simulink model "double_luenberger"  (R2015a)
settings: Solver=ode45  StartTime=0.0  StopTime=3  RelTol=1e-3
PreLoadFcn:
  | double_pend_feedback
InitFcn:
  | double_pend_feedback
StartFcn:
  | double_pend_feedback
values from neighbouring files (symbols this model uses):
  A = [zeros(3,3) eye(3); -inv(D_)*G zeros(3,3)]    [double_pend_feedback.m]    (also in fuzzy_logic.m = [zeros(3,3) eye(3); inv(D_)*G zeros(3,3)]; single_pend.m = [0 1 0 0; (g*(M+m))/(l*M) 0 0 b/(l*M); 0 0 0 1; -m*g/M 0 0 -)
  a = 0.1    [double_pend_feedback.m]    (also in fuzzy_logic.m; single_pend.m)
  A_ = [0 1 0 0; -k/mass -damper/mass (sqrt(ep*2*a*k))/ep*a*mass 0; 0 0 0 1; 0 0 0 -R/L]    [double_pend_feedback.m]    (also in fuzzy_logic.m; single_pend.m)
  B = [zeros(3,1); inv(D_)*H]    [double_pend_feedback.m]    (also in fuzzy_logic.m; single_pend.m = [0;-1/(l*M); 0 ; 1/M])
  B_ = [0; 1/mass; 0;0]    [double_pend_feedback.m]    (also in fuzzy_logic.m; single_pend.m)
  damper = 200    [double_pend_feedback.m]    (also in fuzzy_logic.m; single_pend.m)
  ep = 1    [double_pend_feedback.m]    (also in fuzzy_logic.m; single_pend.m)
  k = 1    [double_pend_feedback.m]    (also in fuzzy_logic.m; single_pend.m)
  K_confirm = acker(A,B,p)    [double_pend_feedback.m]    (also in fuzzy_logic.m)
  Ke_confirm = acker(A',C',pe)    [double_pend_feedback.m]    (also in fuzzy_logic.m)
  L = 0.0001    [double_pend_feedback.m]    (also in fuzzy_logic.m; single_pend.m)
  mass = 0.5    [double_pend_feedback.m]    (also in fuzzy_logic.m; single_pend.m)
  R = 100    [double_pend_feedback.m]    (also in fuzzy_logic.m; single_pend.m)
libraries: simulink x1
settings Model: Creator=Nabeel  LastModifiedBy=Nabeel

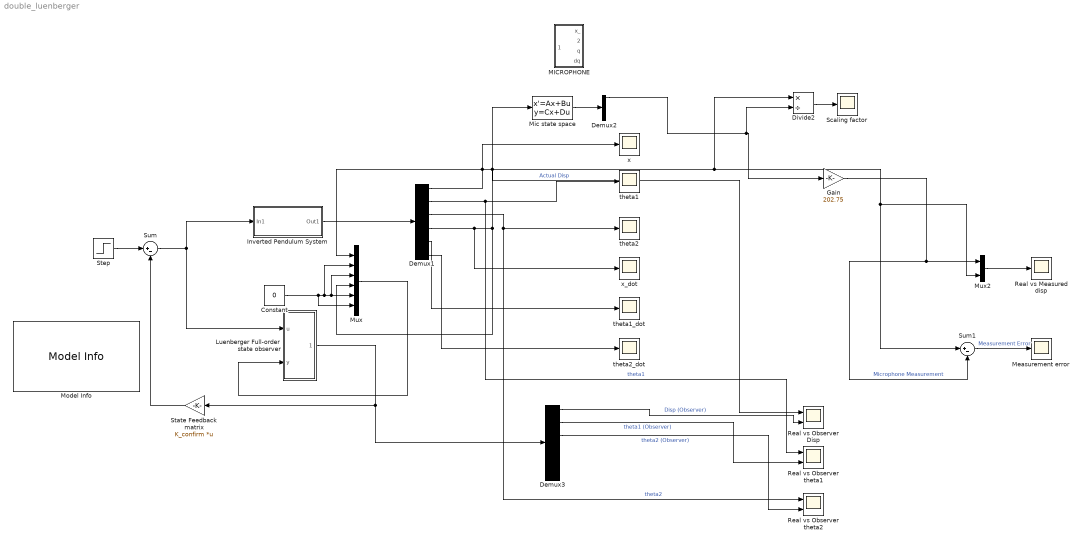
== system double_luenberger ==
  Constant : Constant  Value=0
  Demux1 : Demux  Outputs=6
  Demux2 : Demux
  Demux3 : Demux  Outputs=6
  Divide2 : Product  Inputs=*/
  Gain : Gain  Gain=202.75
  Inverted Pendulum System : Subsystem
  Luenberger Full-order state observer : Subsystem
  MICROPHONE : Subsystem
  Measurement error : Scope
      settings: ShowLegends=on  SaveName=error
  Mic state space : StateSpace  A=A_  B=B_  C=eye(4)  D=[0;0;0;0]  X0=0
  Model Info : simulink/Model-Wide Utilities/Model Info  Frame=on  DisplayStringWithTags=|  HorizontalTextAlignment=Center  LeftAlignmentValue=0.5  SourceBlockDiagram=double_luenberger  TagMaxNumber=20
      | State feedback matrix info:
      | Replace the feedback block
      |  to test other controllers
      | Gain block
      | K- pole placement (non-repeated)
      | lqr1 - LQR 1 as defined in report
      | lqr2- LQR 2 as defined in the report
  Mux : Mux  Inputs=6
  Mux2 : Mux  Inputs=2
  Real vs Measured disp : Scope
      settings: ShowLegends=on  SaveName=mic_v_real
  Real vs Observer Disp : Scope  NumInputPorts=2
      settings: ShowLegends=on  YMin=-425000~-5  YMax=75000~5  SaveName=results
  Real vs Observer theta1 : Scope  NumInputPorts=2
      settings: ShowLegends=on  YMin=-425000~-5  YMax=75000~5  SaveName=results1
  Real vs Observer theta2 : Scope  NumInputPorts=2
      settings: ShowLegends=on  YMin=-425000~-5  YMax=75000~5  SaveName=results2
  Scaling factor : Scope
      settings: ShowLegends=on  SaveName=scaling
  State Feedback matrix : Gain  Gain=K_confirm  Multiplication=Matrix(K*u)
  Step : Step  SampleTime=0
  Sum : Sum  Inputs=|+-
  Sum1 : Sum  Inputs=|+-
  theta1 : Scope
      settings: SaveName=theta1
  theta1_dot : Scope
      settings: SaveName=theta1_dot
  theta2 : Scope
      settings: SaveName=theta2
  theta2_dot : Scope
      settings: SaveName=theta2_dot
  x : Scope
      settings: SaveName=x
  x_dot : Scope
      settings: SaveName=x_dot
  wires:
  Inverted Pendulum System/1(Out1) -> Demux1/1
  Constant/1 -> Mux/6, Mux/2, Mux/3, Mux/5
  Mux/1 -> Luenberger Full-order state observer/2(y)
  Demux1/2 -> theta1/1, Real vs Observer theta1/1  "theta1"
  Demux1/1 -> x/1, Divide2/1, Sum1/1, Mux2/2, Real vs Observer Disp/1, Mux/1  "Actual Disp"
  Mic state space/1 -> Demux2/1
  Step/1 -> Sum/1
  State Feedback matrix/1 -> Sum/2
  Sum/1 -> Inverted Pendulum System/1(In1), Luenberger Full-order state observer/1(u)
  Luenberger Full-order state observer/1(x_estimate) -> Demux3/1, State Feedback matrix/1
  Demux3/1 -> Real vs Observer Disp/2  "Disp (Observer)"
  Demux3/2 -> Real vs Observer theta1/2  "theta1 (Observer)"
  Demux3/3 -> Real vs Observer theta2/2  "theta2 (Observer)"
  Demux1/3 -> theta2/1, Real vs Observer theta2/1  "theta2"
  Gain/1 -> Mux2/1, Sum1/2  "Microphone Measurement"
  Mux2/1 -> Real vs Measured disp/1
  Sum1/1 -> Measurement error/1  "Measurement Error"
  Demux2/1 -> Divide2/2, Gain/1
  Divide2/1 -> Scaling factor/1
  Demux1/5 -> theta1_dot/1
  Demux1/6 -> theta2_dot/1
  Demux1/4 -> x_dot/1, Mic state space/1, Mux/4

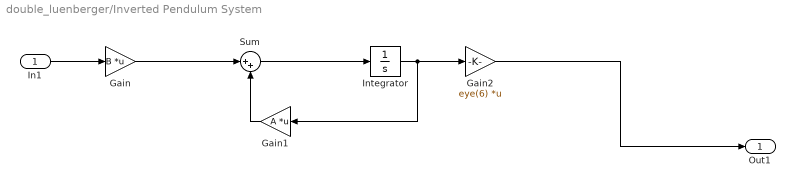
== system double_luenberger/Inverted Pendulum System ==
  In1 : Inport
  Gain : Gain  Gain=B  Multiplication=Matrix(K*u)
  Gain1 : Gain  Gain=A  Multiplication=Matrix(K*u)
  Gain2 : Gain  Gain=eye(6)  Multiplication=Matrix(K*u)
  Integrator : Integrator  InitialCondition=[0 0 0 0 0 0]
  Sum : Sum  Inputs=|++
  Out1 : Outport
  wires:
  In1/1 -> Gain/1
  Gain1/1 -> Sum/2
  Gain/1 -> Sum/1
  Sum/1 -> Integrator/1
  Integrator/1 -> Gain2/1, Gain1/1
  Gain2/1 -> Out1/1

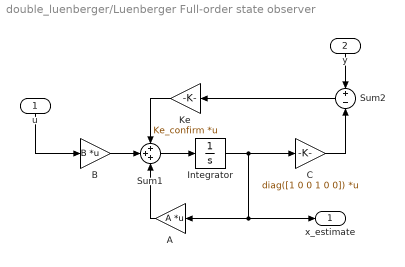
== system double_luenberger/Luenberger Full-order state observer ==
  u : Inport
  y : Inport  Port=2
  A : Gain  Gain=A  Multiplication=Matrix(K*u)
  B : Gain  Gain=B  Multiplication=Matrix(K*u)
  C : Gain  Gain=diag([1 0 0 1 0 0])  Multiplication=Matrix(K*u)
  Integrator : Integrator
  Ke : Gain  Gain=Ke_confirm  Multiplication=Matrix(K*u)
  Sum1 : Sum  Inputs=+++
  Sum2 : Sum  Inputs=+-
  x_estimate : Outport
  wires:
  Sum1/1 -> Integrator/1
  Integrator/1 -> C/1, x_estimate/1, A/1
  Ke/1 -> Sum1/1
  A/1 -> Sum1/3
  B/1 -> Sum1/2
  Sum2/1 -> Ke/1
  y/1 -> Sum2/1
  u/1 -> B/1
  C/1 -> Sum2/2

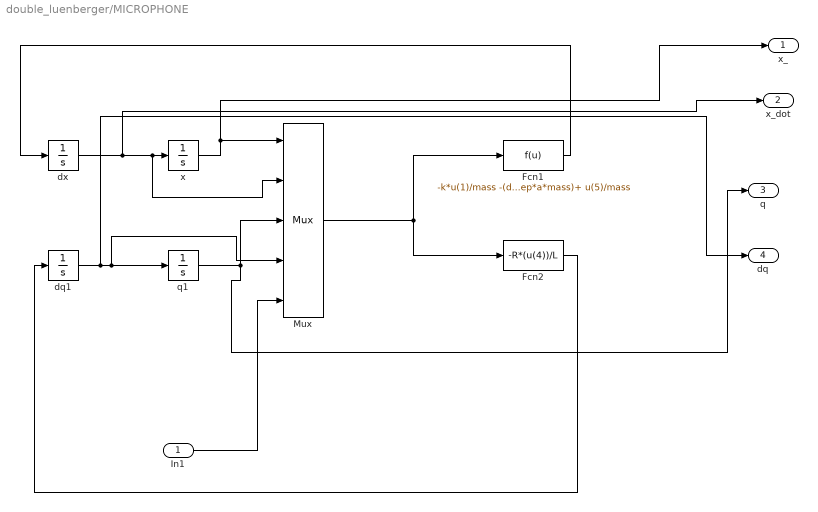
== system double_luenberger/MICROPHONE ==
  In1 : Inport
  Fcn1 : Fcn  Expr=-k*u(1)/mass -(damper*u(2))/mass +(u(3))*((sqrt(ep*2*a*k))/ep*a*mass)+ u(5)/mass
  Fcn2 : Fcn  Expr=-R*(u(4))/L
  Mux : Mux  Inputs=5
  dq1 : Integrator
  dx : Integrator
  q1 : Integrator  InitialCondition=0.01  UpperSaturationLimit=3.14  LowerSaturationLimit=-3.14
  x : Integrator
  x_ : Outport
  x_dot : Outport  Port=2
  q : Outport  Port=3
  dq : Outport  Port=4
  wires:
  Fcn1/1 -> dx/1
  x/1 -> Mux/1, x_/1
  Mux/1 -> Fcn1/1, Fcn2/1
  q1/1 -> q/1, Mux/3
  Fcn2/1 -> dq1/1
  dq1/1 -> Mux/4, q1/1, dq/1
  dx/1 -> x_dot/1, Mux/2, x/1
  In1/1 -> Mux/5
